simulink library "environmentLib"  (R2020b)
settings: Solver=VariableStepAuto  StartTime=0.0  StopTime=10.0  RelTol=1e-3
undefined symbols (not defined in the file): g, rho, States, WMM2020
libraries: aerolibatmos2 x1, aerolibgravity2 x1
settings Model: Creator=dbell44  LastModifiedBy=dbell44

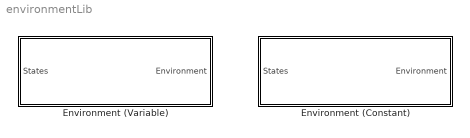
== system environmentLib ==
  Environment (Constant) : Subsystem
  Environment (Variable) : Subsystem

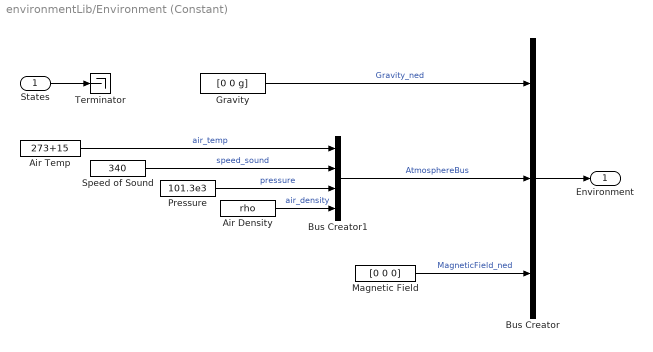
== system environmentLib/Environment (Constant) ==
  States : Inport  OutDataTypeStr=Bus: StatesBus
  Air Density : Constant  Value=rho
  Air Temp : Constant  Value=273+15
  Bus Creator : BusCreator  Inputs=3  OutDataTypeStr=Bus: EnvironmentBus  NonVirtualBus=on
  Bus Creator1 : BusCreator  Inputs=4  OutDataTypeStr=Bus: AtmosphereBus  NonVirtualBus=on
  Gravity : Constant  Value=[0 0 g]
  Magnetic Field : Constant  Value=[0 0 0]
  Pressure : Constant  Value=101.3e3
  Speed of Sound : Constant  Value=340
  Terminator : Terminator
  Environment : Outport  VectorParamsAs1DForOutWhenUnconnected=off
  wires:
  Magnetic Field/1 -> Bus Creator/3  "MagneticField_ned"
  Bus Creator1/1 -> Bus Creator/2  "AtmosphereBus"
  Air Density/1 -> Bus Creator1/4  "air_density"
  Pressure/1 -> Bus Creator1/3  "pressure"
  Speed of Sound/1 -> Bus Creator1/2  "speed_sound"
  Air Temp/1 -> Bus Creator1/1  "air_temp"
  Bus Creator/1 -> Environment/1
  States/1 -> Terminator/1
  Gravity/1 -> Bus Creator/1  "Gravity_ned"

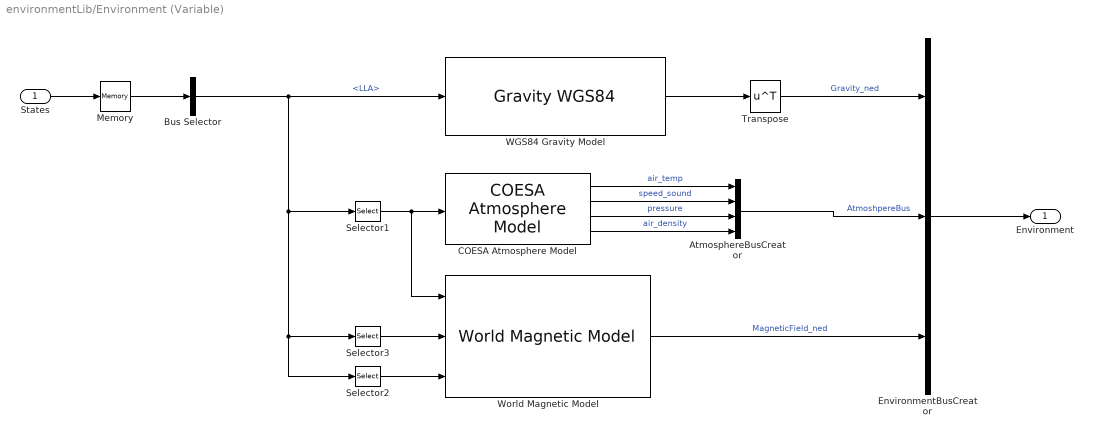
== system environmentLib/Environment (Variable) ==
  States : Inport  OutDataTypeStr=Bus: StatesBus  Interpolate=off
  AtmosphereBusCreator : BusCreator  Inputs=4  OutDataTypeStr=Bus: AtmosphereBus
  Bus Selector : BusSelector  OutputSignals=LLA
  COESA Atmosphere Model : aerolibatmos2/COESA Atmosphere Model  units=Metric (MKS)  spec=1976 COESA-extended U.S. Standard Atmosphere  model=Profile  profile_var=High temperature  profile_percent=1%  profile_alt=5 km (16404 ft)  envelope_var=High temperature  envelope_percent=1%  action=Warning
  EnvironmentBusCreator : BusCreator  Inputs=3  OutDataTypeStr=Bus: EnvironmentBus
  Memory : Memory  InitialCondition=States  InheritSampleTime=on
  Selector1 : Selector  InputPortWidth=3  IndexOptions=Index vector (dialog)  Indices=[3]  OutputSizes=1
  Selector2 : Selector  InputPortWidth=3  IndexOptions=Index vector (dialog)  Indices=[2]  OutputSizes=1
  Selector3 : Selector  InputPortWidth=3  IndexOptions=Index vector (dialog)  Indices=[1]  OutputSizes=1
  Transpose : Math  Operator=transpose  SaturateOnIntegerOverflow=on
  "WGS84 Gravity Model  " : GravityWGS84
  World Magnetic Model : aerolibgravity2/World Magnetic Model  model=WMM2020 (2020-2025)  customFile='WMM2020.COF'  units=Metric (MKS)  time_in=off  month=January  day=1  year=2020  action=Error  h_out=off  dec_out=off  inc_out=off  ti_out=off
      settings: SourceProductBaseCode=AE
  Environment : Outport  OutDataTypeStr=Bus: EnvironmentBus
  wires:
  States/1 -> Memory/1
  COESA Atmosphere Model/1 -> AtmosphereBusCreator/1  "air_temp"
  COESA Atmosphere Model/3 -> AtmosphereBusCreator/3  "pressure"
  World Magnetic Model/1 -> EnvironmentBusCreator/3  "MagneticField_ned"
  Selector3/1 -> World Magnetic Model/2
  EnvironmentBusCreator/1 -> Environment/1
  Bus Selector/1 -> Selector2/1, Selector3/1, Selector1/1, "WGS84 Gravity Model  "/1  "<LLA>"
  "WGS84 Gravity Model  "/1 -> Transpose/1
  Selector1/1 -> COESA Atmosphere Model/1, World Magnetic Model/1
  COESA Atmosphere Model/2 -> AtmosphereBusCreator/2  "speed_sound"
  Memory/1 -> Bus Selector/1
  AtmosphereBusCreator/1 -> EnvironmentBusCreator/2  "AtmoshpereBus"
  COESA Atmosphere Model/4 -> AtmosphereBusCreator/4  "air_density"
  Transpose/1 -> EnvironmentBusCreator/1  "Gravity_ned"
  Selector2/1 -> World Magnetic Model/3
